simulink model "phase2_soc_tool_spike"  (R2026a)
settings: Solver=VariableStepAuto  StopTime=0.15  FixedStep=0.01  EnableMultiTasking=on
undefined symbols (not defined in the file): D1, D2, P
libraries: proctasklib x1
settings Model: Creator=The MathWorks, Inc.  LastModifiedBy=rayyu
settings SolverCC: PositivePriorityOrder=on
settings HardwareCC: ProdBitPerLong=64.0  ProdLargestAtomicInteger=LongLong  ProdLargestAtomicFloat=Double  ProdHWDeviceType=ARM Compatible->ARM Cortex-A (64-bit)  HardwareBoardFeatureSet=SoCBlockset
settings RTWCC: SystemTargetFile=ert.tlc  HardwareBoard=Xilinx Zynq UltraScale+ MPSoC ZCU102 Evaluation Kit  TLCOptions="-aInlineSetEventsForThisBaseRateFcn=TLC_FALSE -aSuppressMultiTaskScheduler=TLC_FALSE  -aRateBasedStepFcn=0"  GenerateReport=on  Toolchain=Linaro AArch64 Linux v6.3.1  IncludeHyperlinkInReport=on  LaunchReport=on  GenerateTraceInfo=on  GenerateTraceReport=on  GenerateTraceReportSl=on  GenerateTraceReportSf=on  GenerateTraceReportEml=on  Description=Embedded Coder
settings ERTTargetCC: ExtModeTransport=2.0  DynamicArrayContainerType=coder::array

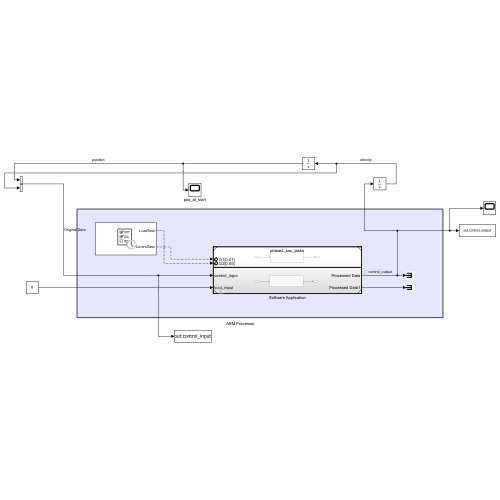
[thumbnail: Simulink's stored preview of the top-level diagram]
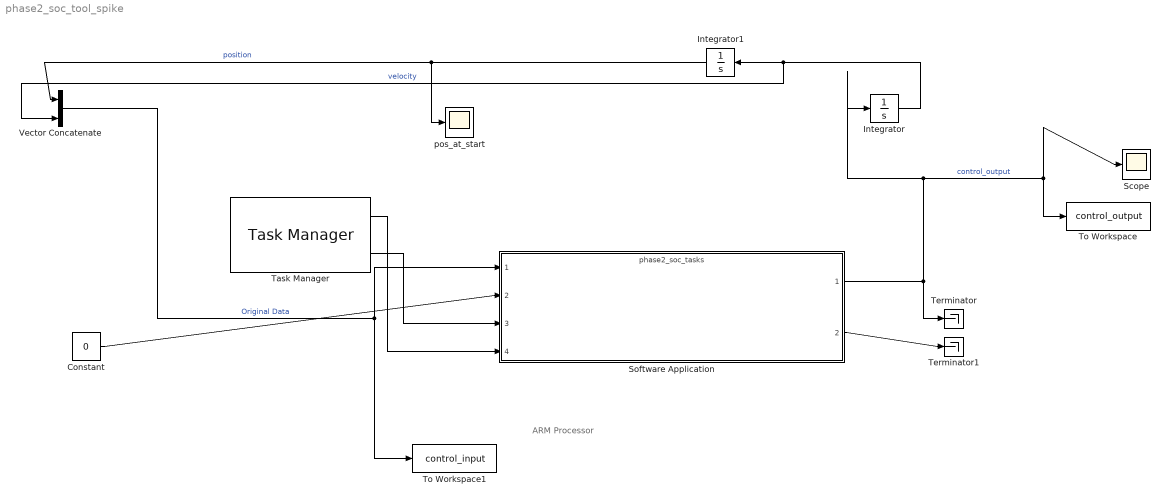
== system phase2_soc_tool_spike ==
  note: ARM Processor
  Constant : Constant  Value=0
  Integrator : Integrator
  Integrator1 : Integrator  InitialCondition=1
  Scope : Scope
      settings: ActiveDisplayYMinimum=-2.25  ActiveDisplayYMaximum=0.24999999999999994
  Software Application : ModelReference  ModelNameDialog=phase2_soc_tasks.slx  SimulationMode=Normal  ScheduleRates=on  CachedPortDiscreteRates=[0.01;0.05]  ModelEventPortInfo=P:D1[0.01][0][0],P:D2[0.05][0][0]  ModelReferenceVersion=14.9
  Task Manager : proctasklib/Task Manager  AllTaskData="[{\"taskName\":\"LoadTask\",\"taskType\":\"Timer-driven\",\"taskEvent\":\"LoadTaskEvent\",\"taskPeriod\":\"0.05\",\"taskPriority\":\"50\",\"coreSelection\":\"Specified core\",\"coreNum\":\"0\",\"dropOverranTasks\":false,\"playbackRecorded\":false,\"diagnosticsFile\":\"\",\"taskDurationSource\":\"Dialog\",\"taskDuration\":1E-6,\"taskDurationDeviation\":0,\"logExecutionData\":true,\"logDroppedTasks\":false,\"version\":\"2.6\",\"taskDurationData\":{\"percent\":\"100\",\"mean\":\"0.03\",\"dev\":\"0\",\"min\":\"0.03\",\"max\":\"0.03\"},\"taskEventSource\":\"Internal\",\"taskEventSourceAssignmentType\":\"AutoAssigned\",\"taskEventSourceType\":\"Unspecified\",\"taskEventGroup\":\"Unspecified\",\"taskEventInterrupt\":\"Unspecified\",\"taskEventOrder\":1,\"taskDisablePremption\":false,\"taskClearInterruptFlagsAtEndOfEvent\":false},{\"taskName\":\"ControlTask\",\"taskType\":\"Timer-driven\",\"taskEvent\":\"ControlTaskEvent\",\"taskPeriod\":\"0.01\",\"taskPriority\":\"50\",\"coreSelection\":\"Specified core\",\"coreNum\":\"0\",\"dropOverranTasks\":false,\"playbackRecorded\":false,\"diagnosticsFile\":\"\",\"taskDurationSource\":\"Dialog\",\"taskDuration\":1E-6,\"taskDurationDeviation\":0,\"logExecutionData\":true,\"logDroppedTasks\":false,\"version\":\"2.6\",\"taskDurationData\":{\"percent\":\"100\",\"mean\":\"0.003\",\"dev\":\"0\",\"min\":\"0.003\",\"max\":\"0.003\"},\"taskEventSource\":\"Internal\",\"taskEventSourceAssignmentType\":\"AutoAssigned\",\"taskEventSourceType\":\"Unspecified\",\"taskEventGroup\":\"Unspecified\",\"taskEventInterrupt\":\"Unspecified\",\"taskEventOrder\":1,\"taskDisablePremption\":false,\"taskClearInterruptFlagsAtEndOfEvent\":false}]"  EnableTaskSimulation=on  StreamToSDI=on  WriteToFile=off  OverwriteFile=off  SupportEventPorts=on  UseScheduleEditor=off  CustomizationInfo=''
  Terminator : Terminator
  Terminator1 : Terminator
  To Workspace : ToWorkspace  VariableName=control_output  SaveFormat=Timeseries  SampleTime=-1
  To Workspace1 : ToWorkspace  VariableName=control_input  SaveFormat=Timeseries  SampleTime=-1
  Vector Concatenate : Concatenate
  pos_at_start : Scope
      settings: ActiveDisplayYMinimum=0.9805911383257554  ActiveDisplayYMaximum=1.0067345814965289
  wires:
  Software Application/1 -> Scope/1, To Workspace/1, Integrator/1, Terminator/1  "control_output"
  Vector Concatenate/1 -> To Workspace1/1, Software Application/1  "Original Data"
  Task Manager/1 -> Software Application/4
  Software Application/2 -> Terminator1/1
  Constant/1 -> Software Application/2
  Integrator/1 -> Vector Concatenate/2, Integrator1/1  "velocity"
  Integrator1/1 -> pos_at_start/1, Vector Concatenate/1  "position"
  Task Manager/2 -> Software Application/3
